simulink model "PDQuadrotor_integrator"  (R2013a)
settings: Solver=ode45  StartTime=0.0  StopTime=10.0  RelTol=1e-3
values from neighbouring files (symbols this model uses):
  b = 3.13*10^(-5)    (= 3.13e-05)    [Quadparameters.m]    (also in dreal_checker.m)
  d = 7.5*10^(-7)    (= 7.5e-07)    [Quadparameters.m]    (also in dreal_checker.m)
  g = 9.81    [Quadparameters.m]    (also in dreal_checker.m)
  Ix = 7.5*10^(-3)    (= 0.0075)    [Quadparameters.m]    (also in dreal_checker.m)
  Iy = 7.5*10^(-3)    (= 0.0075)    [Quadparameters.m]    (also in dreal_checker.m)
  Iz = 1.3*10^(-2)    (= 0.013)    [Quadparameters.m]    (also in dreal_checker.m)
  Jr = 6.5*10^(-5)    (= 6.5e-05)    [Quadparameters.m]    (also in dreal_checker.m)
  l = 0.23    [Quadparameters.m]    (also in dreal_checker.m)
  m = 0.65    [Quadparameters.m]    (also in dreal_checker.m)
settings Model: Creator=abdelrazzak.merheb  LastModifiedBy=merazo
settings DataIOCC: SignalLoggingSaveFormat=ModelDataLogs
settings OptimizationCC: ExpressionDepthLimit=2147483647
settings DebuggingCC: FcnCallInpInsideContextMsg=UseLocalSettings  StrictBusMsg=Warning
settings GRTTargetCC: CombineOutputUpdateFcns=off  GRTInterface=on

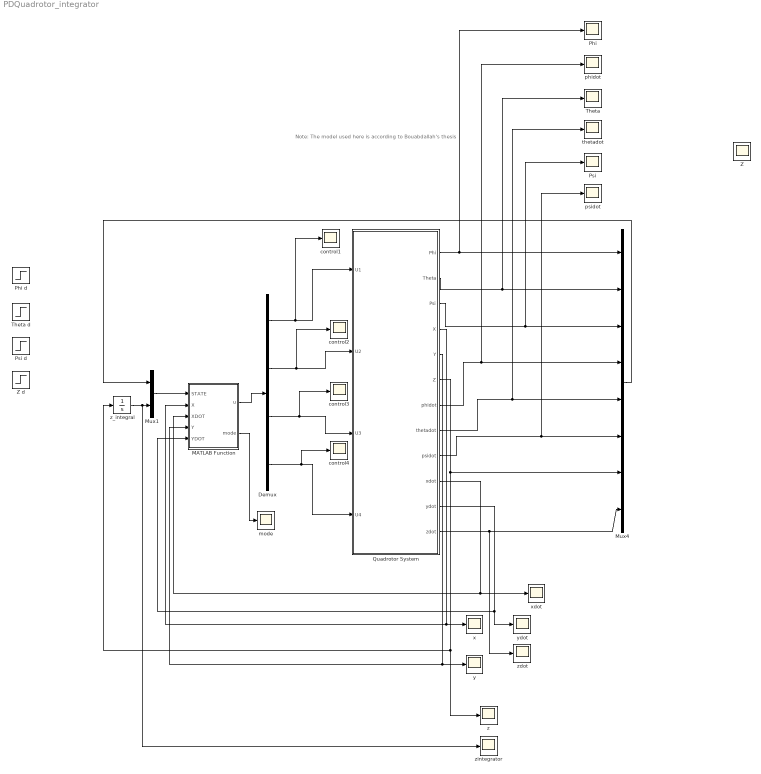
== system PDQuadrotor_integrator ==
  note: Note:
      | The model used here is according to Bouabdallah's thesis
  Demux : Demux
  MATLAB Function : MATLAB Function  TreatAsAtomicUnit=on
  Mux1 : Mux  Inputs=2
  Mux4 : Mux  Inputs=8
  Phi : Scope
  Phi d : Step  SampleTime=0
  Psi : Scope
      settings: SaveName=ScopeData2
  Psi d : Step  SampleTime=0
  Quadrotor System : Subsystem
  Theta : Scope
  Theta d : Step  SampleTime=0
  Z : Scope
      settings: SaveName=ScopeData4
  Z d : Step  SampleTime=0
  "control1 " : Scope
      settings: SaveName=ScopeData14
  control2 : Scope
      settings: SaveName=ScopeData15
  control3 : Scope
      settings: SaveName=ScopeData16
  control4 : Scope
      settings: SaveName=ScopeData17
  mode : Scope
      settings: SaveName=ScopeData19
  phidot : Scope
      settings: SaveName=ScopeData7
  psidot : Scope
      settings: SaveName=ScopeData13
  thetadot : Scope
      settings: SaveName=ScopeData12
  x : Scope
      settings: TimeRange=100  YMin=0  YMax=0.0003  SaveName=ScopeData5
  xdot : Scope
      settings: SaveName=ScopeData9
  y : Scope
      settings: TimeRange=100  YMin=530000  YMax=670000  SaveName=ScopeData3
  ydot : Scope
      settings: SaveName=ScopeData10
  z : Scope
      settings: SaveName=ScopeData8
  z_integral : Integrator  ZeroCross=off
  zdot : Scope
      settings: SaveName=ScopeData11
  zintegrator : Scope
      settings: SaveName=ScopeData18
  wires:
  Quadrotor System/3(Psi) -> Psi/1, Mux4/3
  Quadrotor System/2(Theta) -> Theta/1, Mux4/2
  Quadrotor System/1(Phi) -> Phi/1, Mux4/1
  Demux/2 -> control2/1, Quadrotor System/2(U2)
  Demux/3 -> control3/1, Quadrotor System/3(U3)
  Demux/1 -> "control1 "/1, Quadrotor System/1(U1)
  Demux/4 -> control4/1, Quadrotor System/4(U4)
  MATLAB Function/1(u) -> Demux/1
  Quadrotor System/7(phidot) -> phidot/1, Mux4/4
  Quadrotor System/8(thetadot) -> thetadot/1, Mux4/5
  Quadrotor System/9(psidot) -> psidot/1, Mux4/6
  Quadrotor System/4(X) -> MATLAB Function/2(X), x/1
  Quadrotor System/5(Y) -> MATLAB Function/4(Y), y/1
  Quadrotor System/10(xdot) -> MATLAB Function/3(XDOT), xdot/1
  Quadrotor System/11(ydot) -> MATLAB Function/5(YDOT), ydot/1
  Quadrotor System/12(zdot) -> Mux4/8, zdot/1
  Mux1/1 -> MATLAB Function/1(STATE)
  z_integral/1 -> zintegrator/1, Mux1/2
  Mux4/1 -> Mux1/1
  MATLAB Function/2(mode) -> mode/1
  Quadrotor System/6(Z) -> Mux4/7, z_integral/1, z/1

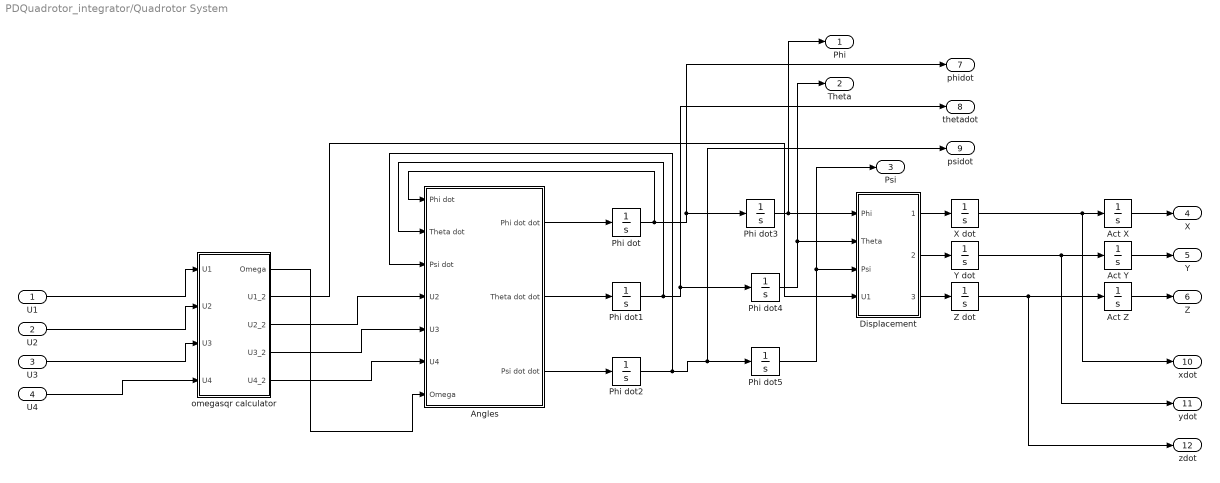
== system PDQuadrotor_integrator/Quadrotor System ==
  U1 : Inport
  U2 : Inport  Port=2
  U3 : Inport  Port=3
  U4 : Inport  Port=4
  Act X : Integrator
  Act Y : Integrator
  Act Z : Integrator
  Angles : Subsystem
  Displacement : Subsystem
  Phi dot : Integrator
  Phi dot1 : Integrator  InitialCondition=0.0  ZeroCross=off
  Phi dot2 : Integrator  ZeroCross=off
  Phi dot3 : Integrator  InitialCondition=0.1  ZeroCross=off
  Phi dot4 : Integrator  ZeroCross=off
  Phi dot5 : Integrator  InitialCondition=0.1  ZeroCross=off
  X dot : Integrator
  Y dot : Integrator
  Z dot : Integrator
  omegasqr calculator : Subsystem
  Phi : Outport
  Theta : Outport  Port=2
  Psi : Outport  Port=3
  X : Outport  Port=4
  Y : Outport  Port=5
  Z : Outport  Port=6
  phidot : Outport  Port=7
  thetadot : Outport  Port=8
  psidot : Outport  Port=9
  xdot : Outport  Port=10
  ydot : Outport  Port=11
  zdot : Outport  Port=12
  wires:
  Angles/1(Phi dot dot) -> Phi dot/1
  Angles/2(Theta dot dot) -> Phi dot1/1
  Angles/3(Psi dot dot) -> Phi dot2/1
  Phi dot/1 -> Angles/1(Phi dot), phidot/1, Phi dot3/1
  Phi dot1/1 -> Angles/2(Theta dot), thetadot/1, Phi dot4/1
  Phi dot2/1 -> Angles/3(Psi dot), psidot/1, Phi dot5/1
  omegasqr calculator/3(U2_2) -> Angles/4(U2)
  omegasqr calculator/4(U3_2) -> Angles/5(U3)
  omegasqr calculator/5(U4_2) -> Angles/6(U4)
  omegasqr calculator/1(Omega) -> Angles/7(Omega)
  Phi dot3/1 -> Displacement/1(Phi), Phi/1
  Phi dot4/1 -> Displacement/2(Theta), Theta/1
  Phi dot5/1 -> Displacement/3(Psi), Psi/1
  omegasqr calculator/2(U1_2) -> Displacement/4(U1)
  Displacement/1(x dotdot) -> X dot/1
  X dot/1 -> xdot/1, Act X/1
  Y dot/1 -> ydot/1, Act Y/1
  Displacement/2(y dotdot) -> Y dot/1
  Z dot/1 -> zdot/1, Act Z/1
  Displacement/3(z dotdot) -> Z dot/1
  Act X/1 -> X/1
  Act Y/1 -> Y/1
  Act Z/1 -> Z/1
  U1/1 -> omegasqr calculator/1(U1)
  U2/1 -> omegasqr calculator/2(U2)
  U3/1 -> omegasqr calculator/3(U3)
  U4/1 -> omegasqr calculator/4(U4)

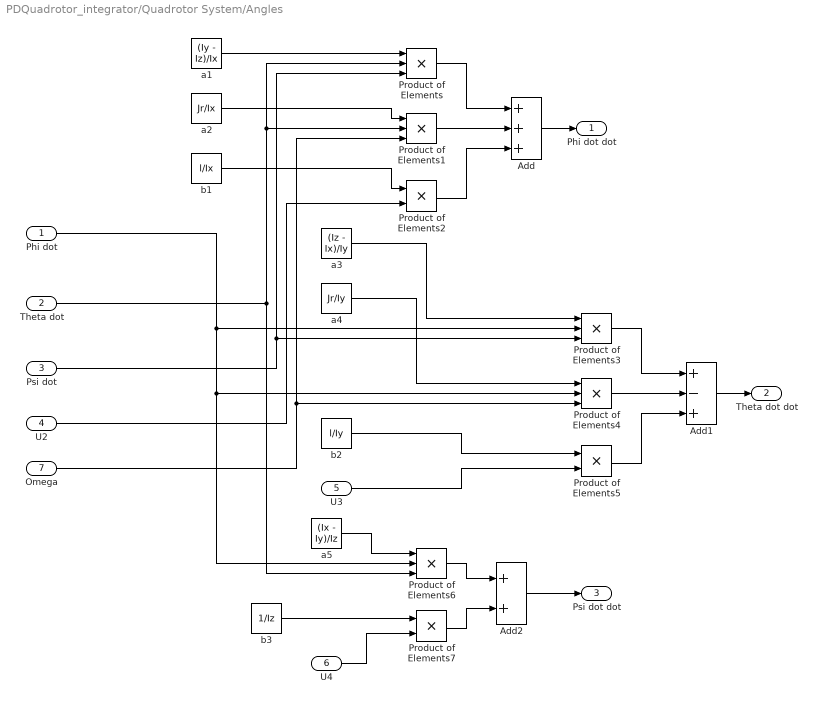
== system PDQuadrotor_integrator/Quadrotor System/Angles ==
  Phi dot : Inport
  Theta dot : Inport  Port=2
  Psi dot : Inport  Port=3
  U2 : Inport  Port=4
  U3 : Inport  Port=5
  U4 : Inport  Port=6
  Omega : Inport  Port=7
  Add : Sum  Inputs=+++
  Add1 : Sum  Inputs=+-+
  Add2 : Sum
  Product of Elements{,1,3..4,6} (5 alike) : Product  Inputs=3
  Product of Elements2 : Product
  Product of Elements5 : Product
  Product of Elements7 : Product
  a1 : Constant  Value=(Iy - Iz)/Ix
  a2 : Constant  Value=Jr/Ix
  a3 : Constant  Value=(Iz - Ix)/Iy
  a4 : Constant  Value=Jr/Iy
  a5 : Constant  Value=(Ix - Iy)/Iz
  b1 : Constant  Value=l/Ix
  b2 : Constant  Value=l/Iy
  b3 : Constant  Value=1/Iz
  Phi dot dot : Outport
  Theta dot dot : Outport  Port=2
  Psi dot dot : Outport  Port=3
  wires:
  Product of Elements/1 -> Add/1
  Product of Elements1/1 -> Add/2
  Product of Elements2/1 -> Add/3
  Add/1 -> Phi dot dot/1
  a1/1 -> Product of Elements/1
  Theta dot/1 -> Product of Elements/2, Product of Elements1/2, Product of Elements6/3
  Psi dot/1 -> Product of Elements/3, Product of Elements3/3
  a2/1 -> Product of Elements1/1
  b1/1 -> Product of Elements2/1
  U2/1 -> Product of Elements2/2
  Omega/1 -> Product of Elements1/3, Product of Elements4/3
  Product of Elements3/1 -> Add1/1
  Product of Elements4/1 -> Add1/2
  Product of Elements5/1 -> Add1/3
  Add1/1 -> Theta dot dot/1
  a3/1 -> Product of Elements3/1
  a4/1 -> Product of Elements4/1
  b2/1 -> Product of Elements5/1
  U3/1 -> Product of Elements5/2
  Phi dot/1 -> Product of Elements3/2, Product of Elements4/2, Product of Elements6/2
  Product of Elements6/1 -> Add2/1
  Product of Elements7/1 -> Add2/2
  Add2/1 -> Psi dot dot/1
  U4/1 -> Product of Elements7/2
  b3/1 -> Product of Elements7/1
  a5/1 -> Product of Elements6/1

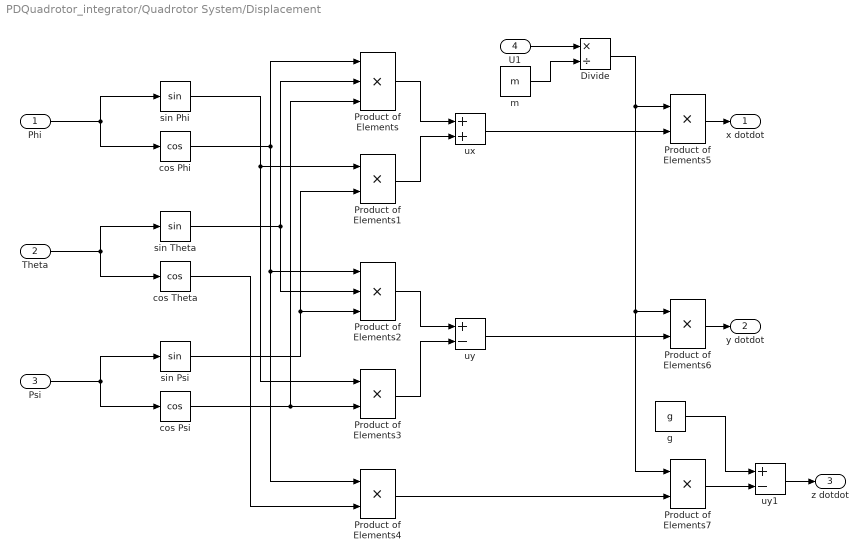
== system PDQuadrotor_integrator/Quadrotor System/Displacement ==
  Phi : Inport
  Theta : Inport  Port=2
  Psi : Inport  Port=3
  U1 : Inport  Port=4
  Divide : Product  Inputs=*/
  Product of Elements : Product  Inputs=3
  Product of Elements{1,3..7} (6 alike) : Product
  Product of Elements2 : Product  Inputs=3
  cos Phi : Trigonometry  Operator=cos
  cos Psi : Trigonometry  Operator=cos
  cos Theta : Trigonometry  Operator=cos
  g : Constant  Value=g
  m : Constant  Value=m
  sin Phi : Trigonometry
  sin Psi : Trigonometry
  sin Theta : Trigonometry
  ux : Sum
  uy : Sum  Inputs=+-
  uy1 : Sum  Inputs=+-
  x dotdot : Outport
  y dotdot : Outport  Port=2
  z dotdot : Outport  Port=3
  wires:
  Phi/1 -> sin Phi/1, cos Phi/1
  Theta/1 -> sin Theta/1, cos Theta/1
  Psi/1 -> sin Psi/1, cos Psi/1
  sin Theta/1 -> Product of Elements/2, Product of Elements2/2
  cos Psi/1 -> Product of Elements/3, Product of Elements3/2
  cos Phi/1 -> Product of Elements/1, Product of Elements2/1, Product of Elements4/1
  sin Phi/1 -> Product of Elements1/1, Product of Elements3/1
  sin Psi/1 -> Product of Elements1/2, Product of Elements2/3
  Product of Elements/1 -> ux/1
  Product of Elements1/1 -> ux/2
  ux/1 -> Product of Elements5/2
  Product of Elements2/1 -> uy/1
  Product of Elements3/1 -> uy/2
  uy/1 -> Product of Elements6/2
  cos Theta/1 -> Product of Elements4/2
  Product of Elements4/1 -> Product of Elements7/2
  U1/1 -> Divide/1
  m/1 -> Divide/2
  Divide/1 -> Product of Elements5/1, Product of Elements6/1, Product of Elements7/1
  Product of Elements5/1 -> x dotdot/1
  Product of Elements6/1 -> y dotdot/1
  uy1/1 -> z dotdot/1
  Product of Elements7/1 -> uy1/2
  g/1 -> uy1/1

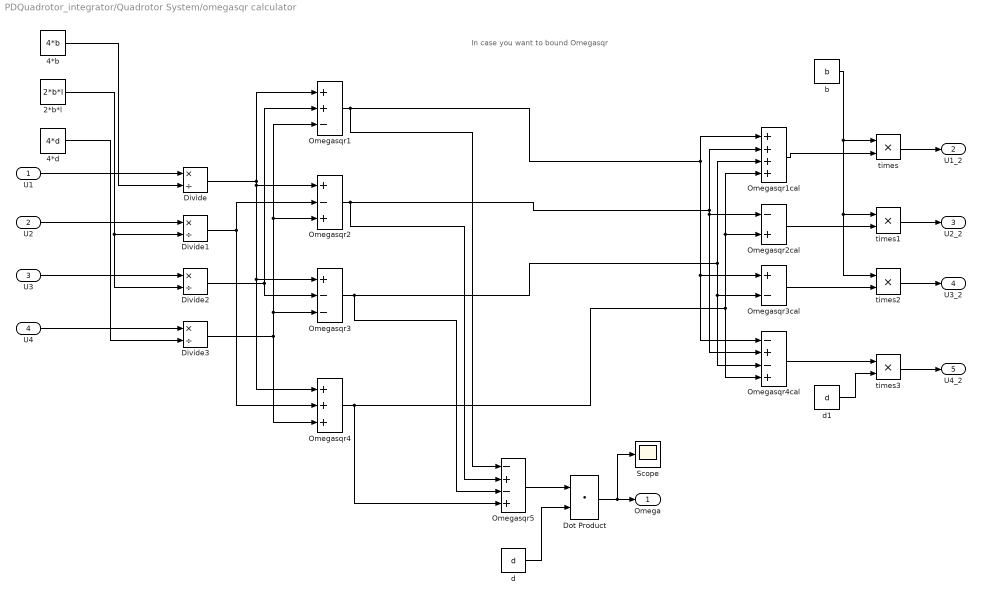
== system PDQuadrotor_integrator/Quadrotor System/omegasqr calculator ==
  note: In case you want to bound Omegasqr
  U1 : Inport
  U2 : Inport  Port=2
  U3 : Inport  Port=3
  U4 : Inport  Port=4
  2*b*l : Constant  Value=2*b*l
  4*b : Constant  Value=4*b
  4*d : Constant  Value=4*d
  Divide{,1..3} (4 alike) : Product  Inputs=*/
  Dot Product : DotProduct  InputSameDT=on  OutDataTypeStr=Inherit: Inherit via internal rule
  Omegasqr1 : Sum  Inputs=++-
  Omegasqr1cal : Sum  Inputs=++++
  Omegasqr2 : Sum  Inputs=+-+
  Omegasqr2cal : Sum  Inputs=-+
  Omegasqr3 : Sum  Inputs=+--
  Omegasqr3cal : Sum  Inputs=+-
  Omegasqr4 : Sum  Inputs=+++
  Omegasqr4cal : Sum  Inputs=-+-+
  Omegasqr5 : Sum  Inputs=-+-+
  Scope : Scope
      settings: SaveName=ScopeData6
  b : Constant  Value=b
  d : Constant  Value=d
  d1 : Constant  Value=d
  times{,1..3} (4 alike) : Product  Inputs=**
  Omega : Outport
  U1_2 : Outport  Port=2
  U2_2 : Outport  Port=3
  U3_2 : Outport  Port=4
  U4_2 : Outport  Port=5
  wires:
  U1/1 -> Divide/1
  4*b/1 -> Divide/2
  U2/1 -> Divide1/1
  2*b*l/1 -> Divide1/2, Divide2/2
  U3/1 -> Divide2/1
  U4/1 -> Divide3/1
  4*d/1 -> Divide3/2
  Divide/1 -> Omegasqr1/1, Omegasqr2/1, Omegasqr3/1, Omegasqr4/1
  Divide2/1 -> Omegasqr1/2, Omegasqr3/2
  Divide3/1 -> Omegasqr1/3, Omegasqr2/3, Omegasqr3/3, Omegasqr4/3
  Divide1/1 -> Omegasqr2/2, Omegasqr4/2
  Omegasqr1/1 -> Omegasqr5/1, Omegasqr1cal/1, Omegasqr3cal/1, Omegasqr4cal/1
  Omegasqr2/1 -> Omegasqr5/2, Omegasqr1cal/2, Omegasqr2cal/1, Omegasqr4cal/2
  Omegasqr3/1 -> Omegasqr5/3, Omegasqr1cal/3, Omegasqr3cal/2, Omegasqr4cal/3
  Omegasqr4/1 -> Omegasqr5/4, Omegasqr1cal/4, Omegasqr2cal/2, Omegasqr4cal/4
  Omegasqr5/1 -> Dot Product/1
  Dot Product/1 -> Scope/1, Omega/1
  d/1 -> Dot Product/2
  b/1 -> times/1, times1/1, times2/1
  Omegasqr1cal/1 -> times/2
  Omegasqr2cal/1 -> times1/2
  Omegasqr3cal/1 -> times2/2
  Omegasqr4cal/1 -> times3/1
  d1/1 -> times3/2
  times/1 -> U1_2/1
  times1/1 -> U2_2/1
  times3/1 -> U4_2/1
  times2/1 -> U3_2/1

== matlab function PDQuadrotor_integrator/MATLAB Function ==
  data: u output; STATE input; X input; XDOT input; Y input; YDOT input; K0 parameter; mode output
function [u, mode] = fcn(STATE, X, XDOT, Y, YDOT, K0)
%#codegen
    kpx = 6;
    kdx = 48;
    kpy = 6;
    kdy = 48;
    u = -K0*(STATE - [kpy*Y + kdy*YDOT; -kpx*X - kdx*XDOT; 0; 0; 0; 0; 0; 0; 0]);
     
 mode = 0;
% u = -K0*STATE;    
%     if ( X >= 0 )
%         u = -K0*(STATE - [0; -kp*X - kd*XDOT; 0; 0; 0; 0; 0; 0; 0]);
%         mode = 1;
%     end
%     
%     if ( X <= -0 )
%         u = -K0*(STATE - [0; -kp*(X) - kd*XDOT; 0; 0; 0; 0; 0; 0; 0]);
%         mode = -1;
%     end
